simulink model "twoTanks_16"  (R2021a)
settings: Solver=ode15s  StartTime=0.0  StopTime=timeFinal  MaxStep=timeStepMax  RelTol=1e-3
undefined symbols (not defined in the file): a1, a2
settings Model: Creator=amit  LastModifiedBy=amit
settings DataIOCC: ExternalInput=ds  LoadExternalInput=on

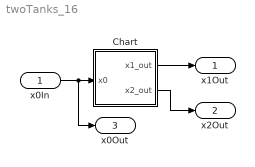
== system twoTanks_16 ==
  x0In : Inport
  Chart : Stateflow chart  TreatAsAtomicUnit=on
  x1Out : Outport  SignalName=x1Out
  x2Out : Outport  Port=2  SignalName=x2Out
  x0Out : Outport  Port=3  SignalName=x0Out
  wires:
  x0In/1 -> Chart/1(x0), x0Out/1
  Chart/2(x2_out) -> x2Out/1
  Chart/1(x1_out) -> x1Out/1

== stateflow chart twoTanks_16/Chart ==
  settings: updateMethod=CONTINUOUS  executeAtInitialization=1
  state loc1
    du:
    x1_dot = 1.0000000 * x0 + -1.0000000 * x1 + 0.0000000 * x2 + -2.0000000 * 1;
    x2_dot = 1.0000000 * x0 + 1.0000000 * x1 + -1.0000000 * x2 + -5.0000000 * 1;
    exit:
    x1_out = x1;
    x2_out = x2;
  state loc2
    du:
    x1_dot = 1.0000000 * x0 + -1.0000000 * x1 + -0.0000000 * x2 + -2.0000000 * 1;
    x2_dot = 1.0000000 * x0 + 1.0000000 * x1 + -0.0000000 * x2 + 0.0000000 * 1;
    exit:
    x1_out = x1;
    x2_out = x2;
  state loc3
    du:
    x1_dot = 1.0000000 * x0 + -1.0000000 * x1 + 0.0000000 * x2 + 3.0000000 * 1;
    x2_dot = 1.0000000 * x0 + 1.0000000 * x1 + -0.0000000 * x2 + -0.0000000 * 1;
    exit:
    x1_out = x1;
    x2_out = x2;
  (default) -> loc1 : {x1 = a1; x2 = a2; }
  (junction 9) -> loc2 : {x1 = x1; x2 = x2; }
  (junction 13) -> loc3 : {x1 = x1; x2 = x2; }
  loc1 -> (junction 5) [order 2]
  (junction 5) -> loc1 : {x1 = x1; x2 = x2; }
  loc2 -> (junction 9) [order 2]
  loc3 -> (junction 13) [order 2]
  loc1 -> loc2 [order 1] : [ 1.0 * x0 + -0.15854571733828515 * x1 + 346.40564835626344 * x2 + -3.408256953048633 * 1 <= 0.000000 + 0]{x1 = 0.0000000 * x0 + 1.0000000 * x1 + 0.0000000 * x2 + 0.000; x2 = 0.0000000 * x0 + 0.0000000 * x1 + 1.0000000 * x2 + 0.000; }
  loc3 -> loc1 [order 1] : [ -8.844818612366703 * x0 + -5.065317516791166 * x1 + -13183.770108019873 * x2 + 13194.47561581206 * 1 <= 0.000000 + 0]{x1 = 0.0000000 * x0 + 1.0000000 * x1 + 0.0000000 * x2 + 0.000; x2 = 0.0000000 * x0 + 0.0000000 * x1 + 1.0000000 * x2 + 0.000; }
  loc2 -> loc3 [order 1] : [ 1.0 * x0 + 4543.3648534226795 * x1 + -0.3834805024612961 * x2 + 4498.02058246409 * 1 <= 0.000000 + 0]{x1 = 0.0000000 * x0 + 1.0000000 * x1 + 0.0000000 * x2 + 0.000; x2 = 0.0000000 * x0 + 0.0000000 * x1 + 1.0000000 * x2 + 0.000; }
  data: x0 input; x1_out output; x2_out output; x1 local double; x2 local double; a1 parameter; a2 parameter
  data x1 settings: updateMethod=SF_CONTINUOUS_TIME_DATA
  data x2 settings: updateMethod=SF_CONTINUOUS_TIME_DATA
